simulink model "solar_tracking_with_PIDcontrol"  (R2021a)
settings: Solver=VariableStepAuto  StartTime=-5  StopTime=30  RelTol=1e-3
model workspace (MAT data in the model file):
  J = 8.6
  Kd = 5
  Kf = 0.07
  Kg = 2000
  Kt = 0.07
  L = 1e-05
  R = 10
libraries: arduinolib x8, pid_lib x1
settings Model: Creator=haider  LastModifiedBy=hufflepuff
settings SolverCC: AlgebraicLoopSolver=TrustRegion
settings DebuggingCC: SFMachineParentedDataDiag=warning

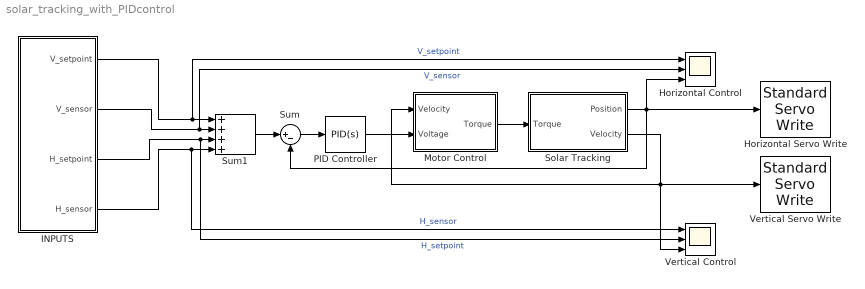
== system solar_tracking_with_PIDcontrol ==
  "Horizontal Control " : Scope  NumInputPorts=3
  Horizontal Servo Write : arduinolib/Standard Servo Write  pinNumber=10  ServoIndex=0  blockPlatform=arduino
  INPUTS : Subsystem
  Motor Control : Subsystem
  PID Controller : pid_lib/PID Controller  Controller=PID  Form=Parallel  TimeDomain=Continuous-time  UseExternalTs=off  SampleTime=-1  IntegratorMethod=Forward Euler  FilterMethod=Forward Euler  ControllerParametersSource=internal  P=320.814393277  I=600.49625354  D=-36.7846486438784  UseFilter=on  N=8.58758696842  TunerSelectOption=Transfer Function Based (PID Tuner App)  InitialConditionSource=internal  InitialConditionForIntegrator=0  InitialConditionForFilter=0  DifferentiatorICPrevScaledInput=0  ExternalReset=none  TrackingMode=off  Kt=1  LimitOutput=off  SatLimitsSource=internal  UpperSaturationLimit=inf  LowerSaturationLimit=-inf  LinearizeAsGain=on  AntiWindupMode=none  Kb=1  POutMin=[]  POutMax=[]  IOutMin=[]  IOutMax=[]  DOutMin=[]  DOutMax=[]  NOutMin=[]  NOutMax=[]  SumOutMin=[]  SumOutMax=[]  SaturationOutMin=[]  SaturationOutMax=[]  PParamMin=[]  PParamMax=[]  IParamMin=[]  IParamMax=[]  DParamMin=[]  DParamMax=[]  NParamMin=[]  NParamMax=[]  KbParamMin=[]  KbParamMax=[]  KtParamMin=[]  KtParamMax=[]  KbOutMin=[]  KbOutMax=[]  KtOutMin=[]  KtOutMax=[]  IntegratorOutMin=[]  IntegratorOutMax=[]  FilterOutMin=[]  FilterOutMax=[]  SumI1OutMin=[]  SumI1OutMax=[]  SumI2OutMin=[]  SumI2OutMax=[]  SumI3OutMin=[]  SumI3OutMax=[]  SumI4OutMin=[]  SumI4OutMax=[]  SumDOutMin=[]  SumDOutMax=[]  DifferentiatorOutMin=[]  DifferentiatorOutMax=[]  FilterDiffOutCoefMin=[]  FilterDiffOutCoefMax=[]  ReciprocalOutMin=[]  ReciprocalOutMax=[]  SumDenOutMin=[]  SumDenOutMax=[]  SumNumOutMin=[]  SumNumOutMax=[]  DivideOutMin=[]  DivideOutMax=[]  UdiffTsProdOutMin=[]  UdiffTsProdOutMax=[]  NTsProdOutMin=[]  NTsProdOutMax=[]  UintegralTsProdOutMin=[]  UintegralTsProdOutMax=[]  UngainTsProdOutMin=[]  UngainTsProdOutMax=[]  IntegratorContinuousStateAttributes=''  IntegratorStateMustResolveToSignalObject=off  IntegratorRTWStateStorageClass=Auto  FilterContinuousStateAttributes=''  FilterStateMustResolveToSignalObject=off  FilterRTWStateStorageClass=Auto  ParallelPVariant=InternalParameters  IdealPVariant=Disabled  IVariant=InternalParameters  DVariant=InternalParameters  IntegratorVariant=Continuous  SatVariant=Disabled  AWVariant=Passthrough  PCopyVariant=Disabled  TRVariant=Disabled  FdbkBlocksVariant=Forward  IdealPFdbkVariant=Disabled  SatFdbkVariant=Disabled  DerivativeFilterVariant=ContFilter  NVariant=InternalParameters  NCopyVariant=Disabled  FilterICVariant=InternalICsFilter  IntegratorICVariant=InternalICs  ExternalResetVariant=Disabled  TRSumVariant=Passthrough  SumFdbkVariant=Disabled  SumVariant=Sum_PID  TsampFilterVariant=InternalTs  TsampNgainVariant=Passthrough  TsampIntegralVariant=Passthrough  ExternalSaturationOutDataTypeStr=Inherit: Same as second input
  Solar Tracking : Subsystem
  Sum : Sum  Inputs=|+-
  Sum1 : Sum  Inputs=+|+|+|+
  "Vertical Control " : Scope  NumInputPorts=3
  Vertical Servo Write : arduinolib/Standard Servo Write  pinNumber=9  ServoIndex=1  blockPlatform=arduino
  wires:
  Solar Tracking/1(Position) -> Sum/2, Horizontal Servo Write/1, "Horizontal Control "/3
  PID Controller/1 -> Motor Control/2(Voltage)
  Motor Control/1(Torque) -> Solar Tracking/1("Torque ")
  Sum/1 -> PID Controller/1
  Sum1/1 -> Sum/1
  INPUTS/3("H_setpoint ") -> "Vertical Control "/2, Sum1/3  "H_setpoint"
  INPUTS/4(H_sensor) -> "Vertical Control "/1, Sum1/4  "H_sensor"
  INPUTS/2(V_sensor) -> "Horizontal Control "/2, Sum1/2  "V_sensor"
  INPUTS/1("V_setpoint ") -> "Horizontal Control "/1, Sum1/1  "V_setpoint"
  Solar Tracking/2(Velocity) -> Motor Control/1(Velocity), Vertical Servo Write/1, "Vertical Control "/3

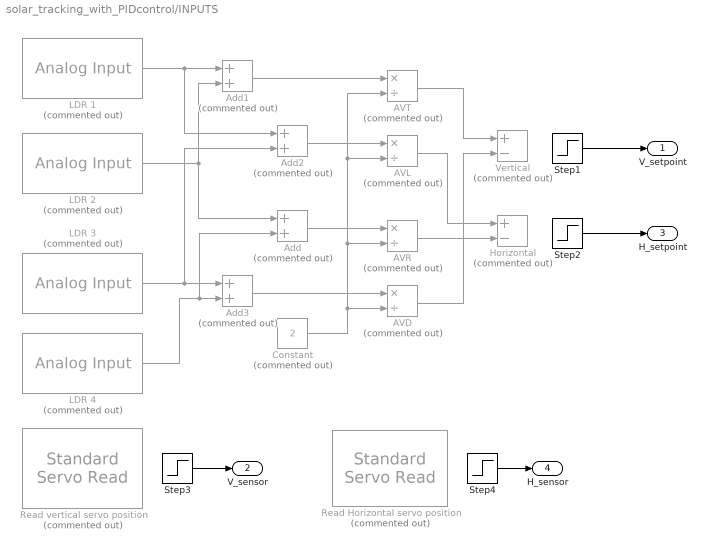
== system solar_tracking_with_PIDcontrol/INPUTS ==
  AVD : Product  Commented=on  Inputs=*/
  AVL : Product  Commented=on  Inputs=*/
  AVR : Product  Commented=on  Inputs=*/
  AVT : Product  Commented=on  Inputs=*/
  Add{,1..3} (4 alike) : Sum  Commented=on
  Constant : Constant  Commented=on  Value=2
  Horizontal : Sum  Commented=on  Inputs=+-
  LDR 1 : arduinolib/Analog Input  Commented=on  pinNumber=0  ReadResultsOnly=off  ConversionTriggerSource=Software  ExternalTriggerType=uint32( 0 )  OutputDataType=uint16  EnableConversionCompleteNotify=off  EnableOuputStatus=off  SampleTime=0.1  blockPlatform=arduino
  LDR 2 : arduinolib/Analog Input  Commented=on  pinNumber=1  ReadResultsOnly=off  ConversionTriggerSource=Software  ExternalTriggerType=uint32( 0 )  OutputDataType=uint16  EnableConversionCompleteNotify=off  EnableOuputStatus=off  SampleTime=0.1  blockPlatform=arduino
  LDR 3 : arduinolib/Analog Input  Commented=on  pinNumber=2  ReadResultsOnly=off  ConversionTriggerSource=Software  ExternalTriggerType=uint32( 0 )  OutputDataType=uint16  EnableConversionCompleteNotify=off  EnableOuputStatus=off  SampleTime=0.1  blockPlatform=arduino
  LDR 4 : arduinolib/Analog Input  Commented=on  pinNumber=3  ReadResultsOnly=off  ConversionTriggerSource=Software  ExternalTriggerType=uint32( 0 )  OutputDataType=uint16  EnableConversionCompleteNotify=off  EnableOuputStatus=off  SampleTime=0.1  blockPlatform=arduino
  Read Horizontal servo position : arduinolib/Standard Servo Read  Commented=on  pinNumber=10  SampleTime=0.1  ServoIndex=0  blockPlatform=arduino
      settings: SourceProductBaseCode=ARDUINO
  Read vertical servo position : arduinolib/Standard Servo Read  Commented=on  pinNumber=9  SampleTime=0.1  ServoIndex=1  blockPlatform=arduino
      settings: SourceProductBaseCode=ARDUINO
  Step{1..4} (4 alike) : Step  Time=0  SampleTime=0
  Vertical : Sum  Commented=on  Inputs=+-
  "V_setpoint " : Outport
  V_sensor : Outport  Port=2
  "H_setpoint " : Outport  Port=3
  H_sensor : Outport  Port=4
  wires:
  LDR 2/1 -> Add/1, Add1/2
  Add2/1 -> AVL/1
  LDR 1/1 -> Add2/1, Add1/1
  AVR/1 -> Horizontal/2
  AVT/1 -> Vertical/1
  LDR 4/1 -> Add/2, Add3/2
  LDR 3/1 -> Add2/2, Add3/1
  Add3/1 -> AVD/1
  AVD/1 -> Vertical/2
  Add/1 -> AVR/1
  Add1/1 -> AVT/1
  Constant/1 -> AVL/2, AVT/2, AVR/2, AVD/2
  AVL/1 -> Horizontal/1
  Step2/1 -> "H_setpoint "/1
  Step3/1 -> V_sensor/1
  Step4/1 -> H_sensor/1
  Step1/1 -> "V_setpoint "/1

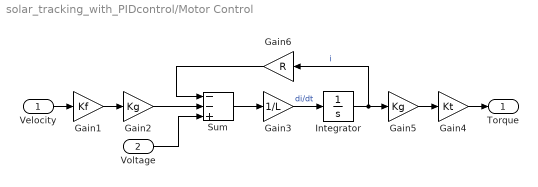
== system solar_tracking_with_PIDcontrol/Motor Control ==
  Velocity : Inport
  Voltage : Inport  Port=2
  Gain1 : Gain  Gain=Kf
  Gain2 : Gain  Gain=Kg
  Gain3 : Gain  Gain=1/L
  Gain4 : Gain  Gain=Kt
  Gain5 : Gain  Gain=Kg
  Gain6 : Gain  Gain=R
  Integrator : Integrator
  Sum : Sum  Inputs=-|-|+
  Torque : Outport
  wires:
  Integrator/1 -> Gain5/1, Gain6/1  "i"
  Velocity/1 -> Gain1/1
  Gain1/1 -> Gain2/1
  Sum/1 -> Gain3/1
  Gain3/1 -> Integrator/1  "di/dt"
  Gain5/1 -> Gain4/1
  Gain4/1 -> Torque/1
  Gain6/1 -> Sum/1
  Gain2/1 -> Sum/2
  Voltage/1 -> Sum/3

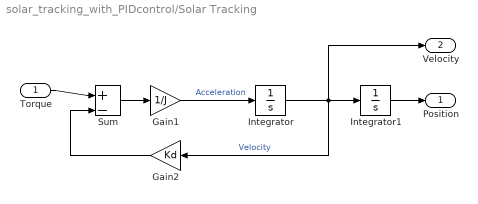
== system solar_tracking_with_PIDcontrol/Solar Tracking ==
  "Torque " : Inport
  Gain1 : Gain  Gain=1/J
  Gain2 : Gain  Gain=Kd
  Integrator : Integrator
  Integrator1 : Integrator
  Sum : Sum  Inputs=+|-
  Position : Outport
  Velocity : Outport  Port=2
  wires:
  Integrator/1 -> Gain2/1, Velocity/1, Integrator1/1  "Velocity"
  Sum/1 -> Gain1/1
  Gain2/1 -> Sum/2
  "Torque "/1 -> Sum/1
  Integrator1/1 -> Position/1
  Gain1/1 -> Integrator/1  "Acceleration"
